simulink model "Drone_NAV_SLAM"  (R2024a)
settings: Solver=FixedStepAuto  StartTime=0.0  StopTime=inf  FixedStep=0.05  RelTol=1e-3
undefined symbols (not defined in the file): DiscIntNeverNeededParam, gray
libraries: robotcorelib x5, mspfiltlib x1, visiongeotforms x1
settings Model: Creator=quentinlandon  LastModifiedBy=quentinlandon
settings SolverCC: AllowMultiTaskInputOutput=on  ConcurrentTasks=on
settings SFSimCC: SimTargetLang=C++

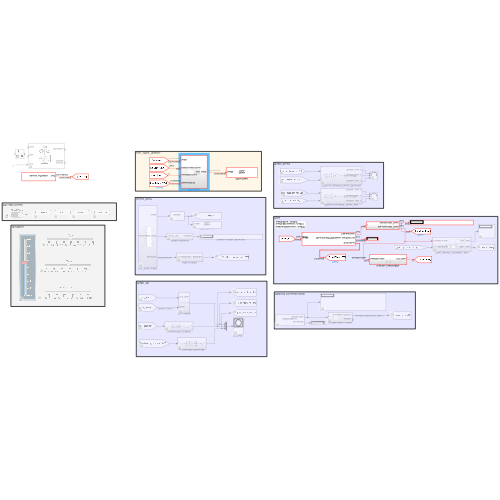
[thumbnail: Simulink's stored preview of the top-level diagram]
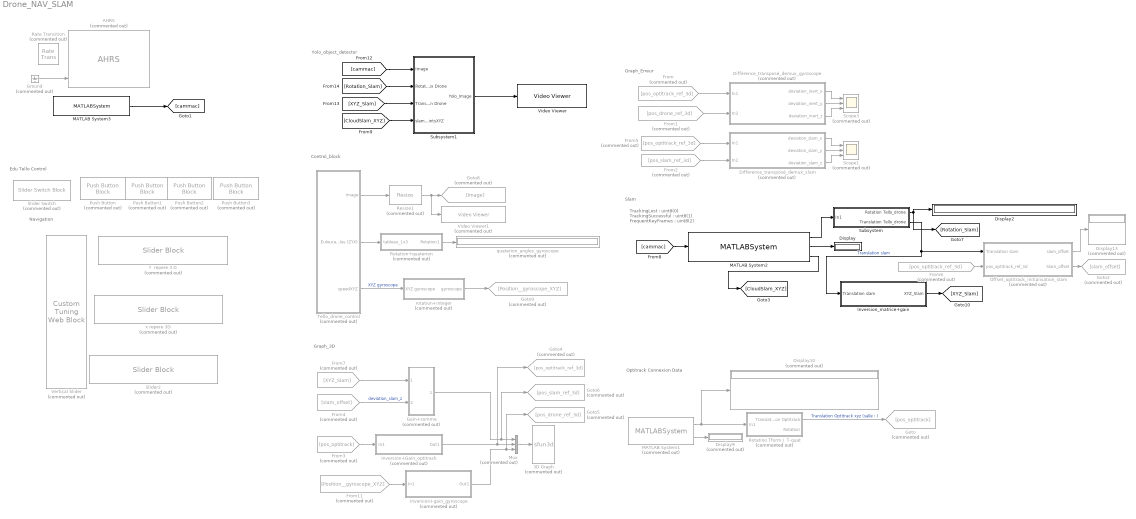
== system Drone_NAV_SLAM ==
  note: Control_block
  note: Graph_Erreur
  note: Graph_3D
  note: Slam
  note: Yolo_object_detector
  note: Optitrack Connexion Data
  note: TrackingLost : uint8(0)
      | TrackingSuccessful : uint8(1)
      | FrequentKeyFrames : uint8(2)
  note: Navigation
  note: Edu Tello Control
  3D Graph : S-Function  Commented=on  LoadFcn=if exist('sfun3d','file'), sfun3d([],[],[],'LoadBlock'); end  FunctionName=sfun3d  Parameters=ax,T,np,cp,gd,ls,mk,mx,hd,tb  SFunctionDeploymentMode=off  EnableBusSupport=off  mask(3D Graph){np=3, ax=[-5 5 -5 5 -5 5], mx=1e4, T=-1, cp=[3 2 1], gd=on, hd=off, tb=on, ls=-, mk=none}
      mask prompts: np "Number of moving points (lines)"; ax "Range: [xmin xmax  ymin ymax zmin zmax]"; mx "Max number of points in each line"; T "Sampling Time"; cp "Camera position (use [0 0 1] for 2D XY view)"; gd "Grid (on|off)"; hd "HeadMarkers (on|off)"; tb "Toolbar (on|off)"; ls "LineStyle"; mk "LineMarker"
      mask help:
      | This block plots the position of several points in the XYZ space. The input contains the coordinates of all the points (x1,y1,z1,x2,y2,z2,...).
      | The number of moving points (lines), the XYZ ranges, sampling time, camera position, and grid (among other things) can be set as mask parameters.
      settings: CopyFcn=if exist('sfun3d','file'), sfun3d([],[],[],'CopyBlock'); end  DeleteFcn=if exist('sfun3d','file'), sfun3d([],[],[],'DeleteBlock'); end  NameChangeFcn=if exist('sfun3d','file'), sfun3d([],[],[],'NameChange'); end
      mask Help:
      | This block plots the position of several points in the XYZ space. The input contains the coordinates of all the points (x1,y1,z1,x2,y2,z2,...).
      | The number of moving points (lines), the XYZ ranges, sampling time, camera position, and grid (among other things) can be set as mask parameters.
      mask TypeOptions ls: - | -- | : | -. | none
      mask TypeOptions mk: none | . | + | o | * | x | square | diamond | v | ^ | > | < | pentagram | hexagram
      mask Display: plot([.05 .95 .95 .05 .05],[.45 .45 .95 .95 .45], 0.5+cos(0:0.1:2*pi)*0.3,0.7+sin(0:0.1:2*pi)*0.2)
  AHRS : mspfiltlib/AHRS  Commented=on  DispRefFrame=NED  DecimationFactor=1  InitialProcessNoise=ahrsfilter.defaultProcessNoise  OrientationFormat=quaternion  SimulateUsing=Interpreted execution  AccelerometerNoise=0.0001924722  GyroscopeNoise=9.1385e-5  MagnetometerNoise=0.1  GyroscopeDriftNoise=3.0462e-13  LinearAccelerationNoise=0.0096236100000000012  MagneticDisturbanceNoise=0.5  LinearAccelerationDecayFactor=0.5  MagneticDisturbanceDecayFactor=0.5  ExpectedMagneticFieldStrength=50
  Différence_transposé_demux_gyroscope : Subsystem  Commented=on
  Différence_transposé_demux_slam : Subsystem  Commented=on
  Display : Display
  Display10 : Display  Commented=on
  Display13 : Display  Commented=on
  Display2 : Display
  Display9 : Display  Commented=on
  From : From  Commented=on  GotoTag=pos_optitrack_ref_3d
  From1 : From  Commented=on  GotoTag=pos_drone_ref_3d
  From11 : From  Commented=on  GotoTag=Position__gyroscope_XYZ
  From2 : From  Commented=on  GotoTag=pos_slam_ref_3d
  From3 : From  Commented=on  GotoTag=pos_optitrack
  From4 : From  Commented=on  GotoTag=slam_offset
  From5 : From  Commented=on  GotoTag=pos_optitrack_ref_3d
  From6 : From  Commented=on  GotoTag=pos_optitrack_ref_3d
  From7 : From  Commented=on  GotoTag=XYZ_Slam
  Gain+somme : Subsystem  Commented=on
  Goto : Goto  Commented=on  GotoTag=pos_optitrack
  Goto2 : Goto  Commented=on  GotoTag=slam_offset
  Goto4 : Goto  Commented=on  GotoTag=pos_optitrack_ref_3d
  Goto5 : Goto  Commented=on  GotoTag=pos_drone_ref_3d
  Goto6 : Goto  Commented=on  GotoTag=pos_slam_ref_3d
  Goto8 : Goto  Commented=on  GotoTag=Image
  Goto9 : Goto  Commented=on  GotoTag=Position__gyroscope_XYZ
  Ground : Ground  Commented=on
  Inversion+Gain_optitrack : Subsystem  Commented=on
  Inversion+gain_gyroscope : Subsystem  Commented=on
  Inversion_matrice+gain : Subsystem
  MATLAB System1 : MATLABSystem  Commented=on  System=OptilinkSystem  HostIP=127.0.0.1  ClientIP=127.0.0.1  SimulateUsing=Interpreted execution
      mask Type: OptilinkSystem
      mask Display:
      | disp('OptilinkSystem');
      | port_label('output',1,'Drones data');
      | port_label('output',2,'Connected');
  MATLAB System2 : MATLABSystem  System=MonoVisualSLAMSystem  FocalLength=[1002.77, 1006.3]  PrincipalPoint=[ 640.67, 365.61 ]  ImageSize=[ 720, 1280 ]  ScaleFactor=1.1  NumLevels=6  MaxNumPoints=1000  SkipMaxFrames=1  TrackFeatureRange=[ 50, 120 ]  LoopClosureThreshold=50  Verbose=false  ThreadLevel=8  SimulateUsing=Interpreted execution
      mask Type: MonoVisualSLAMSystem
      mask Display:
      | disp('MonoVisualSLAMSystem');
      | port_label('input',1,'Image');
      | port_label('output',1,'Camera Pose');
      | port_label('output',2,'Tracking Lost');
      | port_label('output',3,'XYZ Points');
  MATLAB System3 : MATLABSystem  System=camera_ordinateur  SimulateUsing=Interpreted execution
      mask Type: camera_ordinateur
      mask Display:
      | disp('camera_ordinateur');
      | port_label('output',1,'img');
  Mux : Mux  Commented=on  Inputs=3
  Offset_optitrack_initialisation_slam : Subsystem  Commented=on
  Push Button : PushButtonBlock  Commented=on  ButtonText=Takeoff  OffValue=0.000000
  Push Button1 : PushButtonBlock  Commented=on  ButtonText=Land  OffValue=0.000000
  Push Button2 : PushButtonBlock  Commented=on  ButtonText=MoveXYZ  OffValue=0.000000
  Push Button3 : PushButtonBlock  Commented=on  ButtonText=Moverotate  OffValue=0.000000
  Rate Transition : RateTransition  Commented=on
  Resize1 : visiongeotforms/Resize  Commented=on  specify=Output size as a percentage of input size  rfactor=[50 50]  outCols=25  outRows=25  outRowsCols=[25 35]  interp_method=Bilinear  antialias=on  useROI=off  roiFlag=off  roundingMode=Nearest  overflowMode=on  prodOutputMode=Binary point scaling  prodOutputWordLength=32  prodOutputFracLength=10
  Rotatino Tform /  T-quat : Subsystem  Commented=on
  Rotation+quaterion : Subsystem  Commented=on
  Scope1 : Scope  Commented=on  NumInputPorts=3
  Scope3 : Scope  Commented=on  NumInputPorts=3
  Slider Switch : SliderSwitchBlock  Commented=on
      settings: Values={{'Off', 'On'}, [0 1]}
  Slider2 : SliderBlock  Commented=on  ScaleMin=-180  ScaleMax=180
  Subsystem : Subsystem
  Subsystem1 : Subsystem
  Tello_drone_control : Subsystem  Commented=on
  Vertical Slider : CustomTuningWebBlock  Commented=on  LabelPosition=Hide  ShowInitialText=on  Configuration="{\"components\":[{\"name\":\"LinearScaleComponent\",\"settings\":{\"bounds\":{\"max\":2,\"min\":-2,\"tickInterval\":\"auto\"},\"internalTickHeightScaleFactor\":0.5,\"labelColor\":[255,255,200],\"labelFont\":{\"font\":\"Arial\",\"fontSize\":12},\"labelOffset\":0.05,\"labelTransparency\":1,\"needleImage\":{\"size\":[596,842],\"src\":\"data:image\\/svg+xml;base64,PD94bWwgdmVyc2lvbj0iMS4wIiBlbmNvZGluZz0idXRmLTgiPz4NCjwhLS0gR2VuZXJhdG9yOiBBZG9iZSBJbGx1c3RyYXRvciAyNS4wLjAsIFNWRyBFeHBvcnQgUGx1Zy1JbiAuIFNWRyBWZXJzaW9uOiA2LjAwIEJ1aWxkIDApICAtLT4NCjxzdmcgdmVyc2lvbj0iMS4xIg0KCSBpZD0ic3ZnOCIgeG1sbnM6Y2M9Imh0dHA6Ly9jcmVhdGl2ZWNvbW1vbnMub3JnL25zIyIgeG1sbnM6ZGM9Imh0dHA6Ly9wdXJsLm9yZy9kYy9lbGVtZW50cy8xLjEvIiB4bWxuczppbmtzY2FwZT0iaHR0cDovL3d3dy5pbmtzY2FwZS5vcmcvbmFtZXNw ...(+2420 chars)\",\"srcOrientation\":\"horizontal\"},\"needleOffset\":[0.0642123287671233,-0.8044596912521441],\"needleSize\":{\"height\":0.07668067226890757,\"width\":0.4337797619047619},\"position\":[0.03623949579831933,0.2829861111111111,0.6088789682539683,0.9196428571428571],\"referencePoint\":\"auto\",\"scaleColors\":[],\"scaleColorsSize\":0.2,\"scaleDirection\":\"BT\",\"showLabels\":1,\"showMinorTicks\":0,\"showSpanLine\":1,\"showTicks\":1,\"tickColor\":[252,252,197],\"tickTransparency\":1,\"valueBarColor\":[0,114,189],\"valueBarOffset\":-0.27,\"valueBarSize\":0.1,\"valueBarTransparency\":1}},{\"name\":\"BackgroundImageComponent\",\"settings\":{\"image\":{\"size\":[380,101],\"src\":\"data:image\\/svg+xml;base64,PHN2ZyB4bWxucz0iaHR0cDovL3d3dy53My5vcmcvMjAwMC9zdmciIHhtbG5zOnhsaW5rPSJodHRwOi8vd3d3LnczLm9yZy8xOTk5L3hsaW5rIiB2aWV3Qm94PSIwIDAgMzgwIDEwMSI+PGRlZnM+PHN0eWxlPi5jbHMtMXtmaWxsOiMwMDJiNDI7fS5jbHMtMntmaWxsOiM0MjcwODI7fS5jbHMtM3tmaWxsOnVybCgjcmFkaWFsLWdyYWRpZW50KTt9LmNscy00e2ZpbGw6I2M4YzhjODtzdHJva2U6IzAwMDt9PC9zdHlsZT48cmFkaWFsR3JhZGllbnQgaWQ9InJhZGlhbC1ncmFkaWVudCIgY3g9IjE5MCIgY3k9IjUwLjUiIHI9IjI2OS4yMSIgZ3JhZGllbnRVbml0cz0idXNlclNwYWNlT25Vc2UiPjxzdG9wIG9mZnNldD0iMC4wMSIgc3RvcC1jb2xvcj0iIzNlNGY1OCIvPjxzdG9wIG9mZnNldD0iMC4wNiIgc3RvcC1jb2xvcj0iIzQ0NTc2MSIvPjxzdG9wIG9mZnNldD0iMC4xNSIgc3RvcC1jb2xvcj0iIzU1NmE3NiIvPjxzdG9wIG9mZnNldD0iMC4yNSIgc3RvcC1jb2xvcj0iIzZkODg5NSIvPjxzdG9wIG9mZnNldD0iMC4zOCIgc3RvcC1jb2xvcj0iIzhmYjJjMyIvPjxzdG9wIG9mZnNldD0iMC41MiIgc3RvcC1jb2xvcj0iI2I2ZTRmYSIvPjxzdG9wIG9mZnNldD0iMSIgc3RvcC1jb2xvcj0iIzE1NDY1NyIvPjwvcmFkaWFsR3JhZGllbnQ+PC9kZWZzPjxnIGlkPSJmcmFtZSI+PGcgaWQ9IkxheWVyXzIiIGRhdGEtbmFtZT0iTGF5ZXIgMiI+PGcgaWQ9IkxheWVyXzEtMiIgZGF0YS1uYW1lPSJMYXllciAxLTIiPjxyZWN0IGlkPSJyZWN0MTAzNiIgY2xhc3M9ImNscy0xIiB4PSIxMSIgeT0iMTEiIHdpZHRoPSIzNTgiIGhlaWdodD0iNzkiLz48cGF0aCBpZD0icGF0aDEwMzgiIGNsYXNzPSJjbHMtMiIgZD0iTTgsOFY5M0gzNzJWOFpNMzY5LDkwSDExVjExSDM2OVoiLz48cGF0aCBpZD0icGF0aDEwNDAiIGNsYXNzPSJjbHMtMyIgZD0iTTAsMFYxMDFIMzgwVjBaTTM3Miw5M0g4VjhIMzcyWiIvPjwvZz48L2c+PC9nPjxnIGlkPSJ0cmFjayI+PHBhdGggaWQ9InJlY3QxNjExIiBjbGFzcz0iY2xzLTQiIGQ9Ik0zMy4zNywyNi41OUgzNDYuNjNjNCwwLDcuMjUsMi42LDcuMjUsNS44MWgwYzAsMy4yMS0zLjI1LDUuODItNy4yNSw1LjgySDMzLjM3Yy00LDAtNy4yNS0yLjYxLTcuMjUtNS44MmgwQzI2LjEyLDI5LjE5LDI5LjM3LDI2LjU5LDMzLjM3LDI2LjU5WiIvPjwvZz48L3N2Zz4=\",\"srcOrientation\":\"horizontal\"},\"position\":[0,0,1,1],\"scaleMode\":\"0\"}},{\"name\":\"ForegroundImageComponent\",\"settings\":{\"image\":{\"size\":[0,0],\"src\":\"default\",\"srcOrientation\":[]},\"isForeground\":1,\"position\":[0,0,1,1],\"scaleMode\":\"0\"}}],\"settings\":{\"BindingType\":\"param\",\"aspectRatio\":3.7777777777777777,\"backgroundColor\":[0,0,0,\"1\"],\"backgroundOffset\":0,\"backgroundOpacity\":1,\"fixedAspectRatio\":\"on\",\"foregroundColor\":[252,252,196],\"orientation\":\"vertical\",\"showBackgroundColor\":false,\"value\":0,\"version\":\"R2023a\"},\"type\":\"LinearGauge\"}"
  Video Viewer : VideoViewer  colormapValue=gray(256)  FigPos=[1 642 730 455]
  Video Viewer1 : VideoViewer  Commented=on  FigPos=[269 662 902 426]
  Y  repere 3 D : SliderBlock  Commented=on  ScaleMin=-2  ScaleMax=2
  quaterion_angles_gyroscope : Display  Commented=on
  rotation+integer : Subsystem  Commented=on
  x repere 3D : SliderBlock  Commented=on  ScaleMin=-2  ScaleMax=2
  wires:
  MATLAB System2/2 -> Display/1
  Subsystem/1(Rotation Tello_drone) -> Display2/1, [Rotation_Slam]
  MATLAB System1/2 -> Display9/1
  MATLAB System1/1 -> Display10/1, Rotatino Tform /  T-quat/1(In1)
  Subsystem/2(Translation Tello_drone) -> Offset_optitrack_initialisation_slam/1(Translation slam), Inversion_matrice+gain/1(Translation slam)  "Translation slam"
  Tello_drone_control/3(speedXYZ) -> rotation+integer/1(XYZ gyroscope)  "XYZ gyroscope"
  Rotatino Tform /  T-quat/1(Translation Optitrack) -> Goto/1  "Translation Optitrack xyz (salle : )"
  Tello_drone_control/2(Euleurangles (ZYX)) -> Rotation+quaterion/1(tableau_1x3)
  Rotation+quaterion/1(Rotation1) -> quaterion_angles_gyroscope/1
  Resize1/1 -> Goto8/1, Video Viewer1/1
  Tello_drone_control/1(Image) -> Resize1/1
  rotation+integer/1(gyroscope) -> Goto9/1
  Offset_optitrack_initialisation_slam/1(slam_offset) -> Display13/1
  Inversion_matrice+gain/1(XYZ_Slam) -> [XYZ_Slam]
  Offset_optitrack_initialisation_slam/2(Slam_offset) -> Goto2/1
  From6/1 -> Offset_optitrack_initialisation_slam/2(pos_optitrack_ref_3d)
  Mux/1 -> 3D Graph/1
  MATLAB System2/1 -> Subsystem/1(In1)
  Ground/1 -> AHRS/3
  From7/1 -> Gain+somme/1(XYZ_Slam)
  From4/1 -> Gain+somme/2(Offset)  "deviation_slam_z"
  Inversion+Gain_optitrack/1(Out1) -> Goto4/1, Mux/2
  From3/1 -> Inversion+Gain_optitrack/1(In1)
  Inversion+gain_gyroscope/1(Out1) -> Goto5/1, Mux/3
  From11/1 -> Inversion+gain_gyroscope/1(In1)
  Gain+somme/1(Out1) -> Goto6/1, Mux/1
  From/1 -> Différence_transposé_demux_gyroscope/1(In1)
  From1/1 -> Différence_transposé_demux_gyroscope/2(In2)
  Différence_transposé_demux_gyroscope/1(deviation_inert_x) -> Scope3/1
  Différence_transposé_demux_gyroscope/2(deviation_inert_y) -> Scope3/2
  Différence_transposé_demux_gyroscope/3(deviation_inert_z) -> Scope3/3
  From5/1 -> Différence_transposé_demux_slam/1(In1)
  From2/1 -> Différence_transposé_demux_slam/2(In2)
  Différence_transposé_demux_slam/1(deviation_slam_x) -> Scope1/1
  Différence_transposé_demux_slam/2(deviation_slam_y) -> Scope1/2
  Différence_transposé_demux_slam/3(deviation_slam_z) -> Scope1/3
  [cammac] -> MATLAB System2/1
  MATLAB System3/1 -> [cammac]
  Subsystem1/1(Yolo_Image) -> Video Viewer/1
  [cammac] -> Subsystem1/1(Image)
  [XYZ_Slam] -> Subsystem1/3(Translation Drone)
  [Rotation_Slam] -> Subsystem1/2(Rotation matrix Drone)
  MATLAB System2/3 -> [CloudSlam_XYZ]
  [CloudSlam_XYZ] -> Subsystem1/4(slamPointsXYZ)

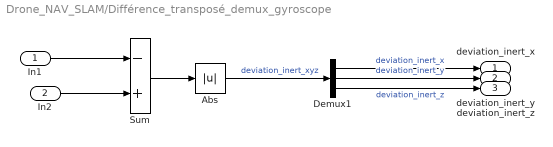
== system Drone_NAV_SLAM/Différence_transposé_demux_gyroscope ==
  In1 : Inport
  In2 : Inport  Port=2
  Abs : Abs  SaturateOnIntegerOverflow=off
  Demux1 : Demux  Outputs=3
  Sum : Sum  Inputs=-+
  deviation_inert_x : Outport
  deviation_inert_y : Outport  Port=2
  deviation_inert_z : Outport  Port=3
  wires:
  Demux1/3 -> deviation_inert_z/1  "deviation_inert_z"
  Demux1/2 -> deviation_inert_y/1  "deviation_inert_y"
  In2/1 -> Sum/2
  In1/1 -> Sum/1
  Demux1/1 -> deviation_inert_x/1  "deviation_inert_x"
  Abs/1 -> Demux1/1  "deviation_inert_xyz"
  Sum/1 -> Abs/1

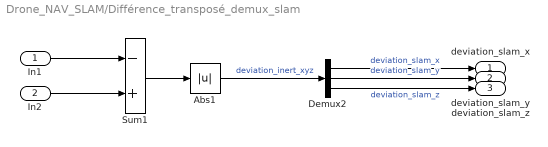
== system Drone_NAV_SLAM/Différence_transposé_demux_slam ==
  In1 : Inport
  In2 : Inport  Port=2
  Abs1 : Abs  SaturateOnIntegerOverflow=off
  Demux2 : Demux  Outputs=3
  Sum1 : Sum  Inputs=-+
  deviation_slam_x : Outport
  deviation_slam_y : Outport  Port=2
  deviation_slam_z : Outport  Port=3
  wires:
  In1/1 -> Sum1/1
  Demux2/1 -> deviation_slam_x/1  "deviation_slam_x"
  In2/1 -> Sum1/2
  Demux2/3 -> deviation_slam_z/1  "deviation_slam_z"
  Abs1/1 -> Demux2/1  "deviation_inert_xyz"
  Sum1/1 -> Abs1/1
  Demux2/2 -> deviation_slam_y/1  "deviation_slam_y"

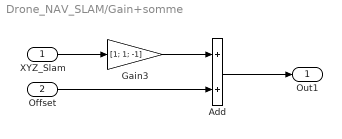
== system Drone_NAV_SLAM/Gain+somme ==
  XYZ_Slam : Inport
  Offset : Inport  Port=2
  Add : Sum
  Gain3 : Gain  Gain=[1; 1; -1]
  Out1 : Outport
  wires:
  XYZ_Slam/1 -> Gain3/1
  Offset/1 -> Add/2
  Add/1 -> Out1/1
  Gain3/1 -> Add/1

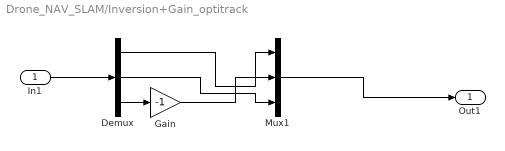
== system Drone_NAV_SLAM/Inversion+Gain_optitrack ==
  In1 : Inport
  Demux : Demux  Outputs=3
  Gain : Gain  Gain=-1
  Mux1 : Mux  Inputs=3
  Out1 : Outport
  wires:
  Mux1/1 -> Out1/1
  Demux/3 -> Gain/1
  Demux/2 -> Mux1/3
  In1/1 -> Demux/1
  Demux/1 -> Mux1/1
  Gain/1 -> Mux1/2

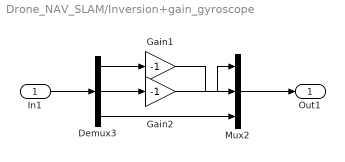
== system Drone_NAV_SLAM/Inversion+gain_gyroscope ==
  In1 : Inport
  Demux3 : Demux  Outputs=3
  Gain1 : Gain  Gain=-1
  Gain2 : Gain  Gain=-1
  Mux2 : Mux  Inputs=3
  Out1 : Outport
  wires:
  In1/1 -> Demux3/1
  Mux2/1 -> Out1/1
  Demux3/1 -> Gain1/1
  Demux3/3 -> Mux2/3
  Gain1/1 -> Mux2/2
  Demux3/2 -> Gain2/1
  Gain2/1 -> Mux2/1

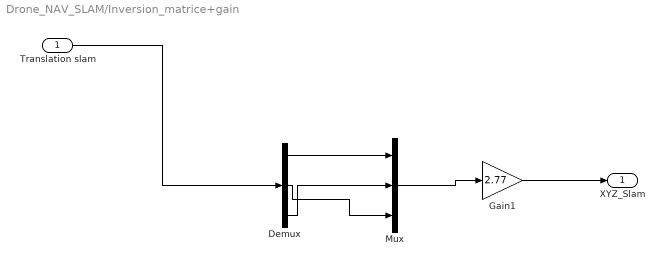
== system Drone_NAV_SLAM/Inversion_matrice+gain ==
  Translation slam : Inport
  Demux : Demux  Outputs=3
  Gain1 : Gain  Gain=2.77
  Mux : Mux  Inputs=3
  XYZ_Slam : Outport
  wires:
  Translation slam/1 -> Demux/1
  Gain1/1 -> XYZ_Slam/1
  Demux/1 -> Mux/1
  Demux/3 -> Mux/2
  Demux/2 -> Mux/3
  Mux/1 -> Gain1/1

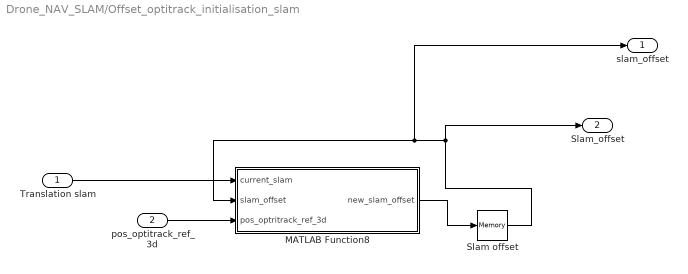
== system Drone_NAV_SLAM/Offset_optitrack_initialisation_slam ==
  Translation slam : Inport
  pos_optitrack_ref_3d : Inport  Port=2
  MATLAB Function8 : MATLAB Function  TreatAsAtomicUnit=on
  Slam offset : Memory  InitialCondition=[0;0;0]
  slam_offset : Outport
  Slam_offset : Outport  Port=2
  wires:
  MATLAB Function8/1(new_slam_offset) -> Slam offset/1
  Slam offset/1 -> Slam_offset/1, slam_offset/1, MATLAB Function8/2(slam_offset)
  Translation slam/1 -> MATLAB Function8/1(current_slam)
  pos_optitrack_ref_3d/1 -> MATLAB Function8/3(pos_optritrack_ref_3d)

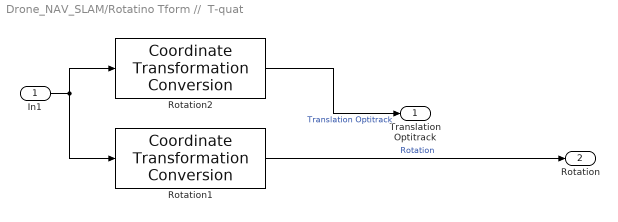
== system Drone_NAV_SLAM/Rotatino Tform //  T-quat ==
  In1 : Inport
  Rotation1 : robotcorelib/Coordinate Transformation Conversion  InputRepresentation=Homogeneous Transformation  InputEulerSequence=ZYX  ShowTrVecInputPort=on  OutputRepresentation=Quaternion  OutputEulerSequence=ZYX  ShowTrVecOutputPort=off  SimulateUsing=Code generation
      settings: LibrarySourceBlock=uavutilslib/Coordinate Transformation Conversion
  Rotation2 : robotcorelib/Coordinate Transformation Conversion  InputRepresentation=Homogeneous Transformation  InputEulerSequence=ZYX  ShowTrVecInputPort=on  OutputRepresentation=Translation Vector  OutputEulerSequence=ZYX  ShowTrVecOutputPort=off  SimulateUsing=Code generation
      settings: LibrarySourceBlock=uavutilslib/Coordinate Transformation Conversion
  Translation Optitrack : Outport
  Rotation : Outport  Port=2
  wires:
  Rotation1/1 -> Rotation/1  "Rotation"
  Rotation2/1 -> Translation Optitrack/1  "Translation Optitrack"
  In1/1 -> Rotation2/1, Rotation1/1

== system Drone_NAV_SLAM/Rotation+quaterion ==
  tableau_1x3 : Inport
  Rotation : robotcorelib/Coordinate Transformation Conversion  InputRepresentation=Euler Angles  InputEulerSequence=ZYX  ShowTrVecInputPort=on  OutputRepresentation=Quaternion  OutputEulerSequence=ZYX  ShowTrVecOutputPort=off  SimulateUsing=Code generation
      settings: LibrarySourceBlock=uavutilslib/Coordinate Transformation Conversion
  Transpose : Math  Operator=transpose
  Rotation1 : Outport
  wires:
  Rotation/1 -> Rotation1/1  "Rotation"
  Transpose/1 -> Rotation/1
  tableau_1x3/1 -> Transpose/1

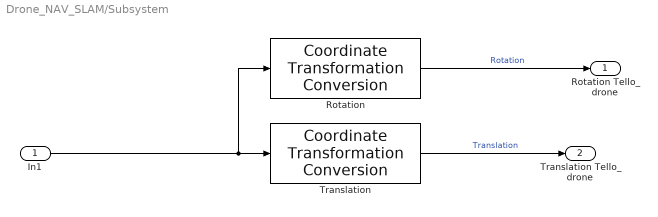
== system Drone_NAV_SLAM/Subsystem ==
  In1 : Inport
  Rotation : robotcorelib/Coordinate Transformation Conversion  InputRepresentation=Homogeneous Transformation  InputEulerSequence=ZYX  ShowTrVecInputPort=on  OutputRepresentation=Rotation Matrix  OutputEulerSequence=ZYX  ShowTrVecOutputPort=off  SimulateUsing=Code generation
      settings: LibrarySourceBlock=uavutilslib/Coordinate Transformation Conversion
  Translation : robotcorelib/Coordinate Transformation Conversion  InputRepresentation=Homogeneous Transformation  InputEulerSequence=ZYX  ShowTrVecInputPort=on  OutputRepresentation=Translation Vector  OutputEulerSequence=ZYX  ShowTrVecOutputPort=on  SimulateUsing=Code generation
      settings: LibrarySourceBlock=uavutilslib/Coordinate Transformation Conversion
  Rotation Tello_drone : Outport
  Translation Tello_drone : Outport  Port=2
  wires:
  Translation/1 -> Translation Tello_drone/1  "Translation"
  Rotation/1 -> Rotation Tello_drone/1  "Rotation"
  In1/1 -> Rotation/1, Translation/1

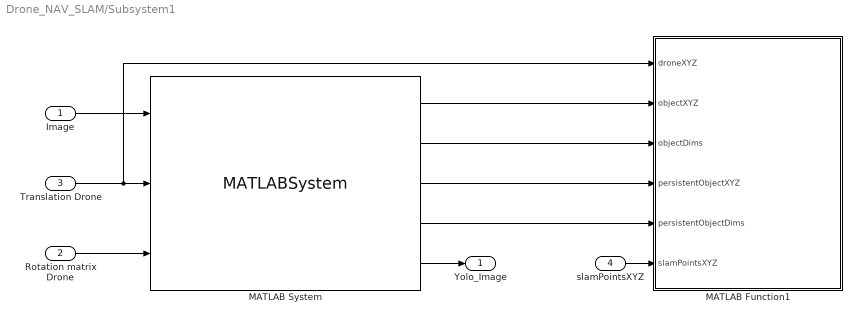
== system Drone_NAV_SLAM/Subsystem1 ==
  Image : Inport
  Rotation matrix Drone : Inport  Port=2
  Translation Drone : Inport  Port=3
  slamPointsXYZ : Inport  Port=4
  MATLAB Function1 : MATLAB Function  TreatAsAtomicUnit=on
  MATLAB System : MATLABSystem  System=Yolo_Object_Detector  SimulateUsing=Interpreted execution
      mask Type: Yolo_Object_Detector
      mask Display:
      | disp('Yolo_Object_Detector');
      | port_label('input',1,'Image');
      | port_label('input',2,'TranslationMatrix');
      | port_label('input',3,'RotationMatrix');
      | port_label('output',1,'ObjectXYZ');
      | port_label('output',2,'ObjectDims');
      | port_label('output',3,'PersistentObjectXYZ');
      | port_label('output',4,'PersistentObjectDims');
      | port_label('output',5,'AnnotatedImage');
  Yolo_Image : Outport
  wires:
  Image/1 -> MATLAB System/1
  Translation Drone/1 -> MATLAB Function1/1(droneXYZ), MATLAB System/2
  MATLAB System/3 -> MATLAB Function1/4(persistentObjectXYZ)
  MATLAB System/4 -> MATLAB Function1/5(persistentObjectDims)
  MATLAB System/2 -> MATLAB Function1/3(objectDims)
  slamPointsXYZ/1 -> MATLAB Function1/6(slamPointsXYZ)
  MATLAB System/5 -> Yolo_Image/1
  Rotation matrix Drone/1 -> MATLAB System/3
  MATLAB System/1 -> MATLAB Function1/2(objectXYZ)

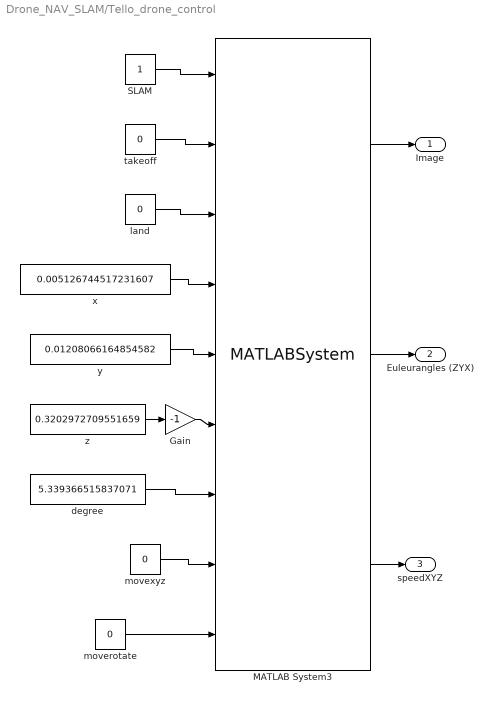
== system Drone_NAV_SLAM/Tello_drone_control ==
  Gain : Gain  Gain=-1
  MATLAB System3 : MATLABSystem  System=Tello_drone_control  droneIP=193.169.0.11  SimulateUsing=Interpreted execution
      mask Type: Tello_drone_control
      mask Display:
      | disp('Tello_drone_control');
      | port_label('input',1,'Slam');
      | port_label('input',2,'tkoff');
      | port_label('input',3,'landing');
      | port_label('input',4,'xMove');
      | port_label('input',5,'yMove');
      | port_label('input',6,'zMove');
      | port_label('input',7,'degree');
      | port_label('input',8,'movexyz');
      | port_label('input',9,'moverotate');
      | port_label('output',1,'imgresize');
      | port_label('output',2,'Eulerangles');
      | port_label('output',3,'speedXYZ');
  SLAM : Constant
  degree : Constant  Value=5.339366515837071
  land : Constant  Value=0
  moverotate : Constant  Value=0
  movexyz : Constant  Value=0
  takeoff : Constant  Value=0
  x : Constant  Value=0.005126744517231607
  y : Constant  Value=0.01208066164854582
  z : Constant  Value=0.3202972709551659
  Image : Outport
  Euleurangles (ZYX) : Outport  Port=2
  speedXYZ : Outport  Port=3
  wires:
  moverotate/1 -> MATLAB System3/9
  land/1 -> MATLAB System3/3
  y/1 -> MATLAB System3/5
  x/1 -> MATLAB System3/4
  Gain/1 -> MATLAB System3/6
  z/1 -> Gain/1
  degree/1 -> MATLAB System3/7
  SLAM/1 -> MATLAB System3/1
  movexyz/1 -> MATLAB System3/8
  MATLAB System3/1 -> Image/1
  takeoff/1 -> MATLAB System3/2
  MATLAB System3/2 -> Euleurangles (ZYX)/1
  MATLAB System3/3 -> speedXYZ/1

== system Drone_NAV_SLAM/rotation+integer ==
  XYZ gyroscope : Inport
  Discrete-Time Integrator : DiscreteIntegrator  SampleTime=-1  ICPrevOutput=DiscIntNeverNeededParam  ICPrevScaledInput=DiscIntNeverNeededParam
  Transpose : Math  Operator=transpose
  gyroscope : Outport
  wires:
  XYZ gyroscope/1 -> Discrete-Time Integrator/1
  Transpose/1 -> gyroscope/1  "gyroscope"
  Discrete-Time Integrator/1 -> Transpose/1

== matlab function Drone_NAV_SLAM/Subsystem1/MATLAB Function1 ==
  data: droneXYZ input; objectXYZ input; objectDims input; persistentObjectXYZ input; persistentObjectDims input; slamPointsXYZ input
function plotCubes(droneXYZ, objectXYZ, objectDims, persistentObjectXYZ, persistentObjectDims, slamPointsXYZ)
    %#codegen
    coder.extrinsic('figure', 'clf', 'hold', 'patch', 'xlabel', 'ylabel', 'zlabel', 'grid', 'axis', 'title', 'view', 'xlim', 'ylim', 'zlim');
    
    %% Initialisation de la figure
    fig = figure(1);
    clf(fig); % Effacer la figure courante
    hold on;
    
    %% Tracer la position du drone
    plot3(droneXYZ(1), droneXYZ(2), droneXYZ(3), 'ro', 'MarkerSize', 10, 'LineWidth', 2);
    
    %% Tracer les objets détectés
    for i = 1:size(objectXYZ, 1)
        if all(objectXYZ(i, :) ~= 0)
            plotBox3D(objectXYZ(i, :), objectDims(i, :), [1, 0, 0], 0.3);
        end
    end
    
    %% Tracer les objets persistants
    for i = 1:size(persistentObjectXYZ, 1)
        if all(persistentObjectXYZ(i, :) ~= 0)
            plotBox3D(persistentObjectXYZ(i, :), persistentObjectDims(i, :), [0, 1, 0], 0.3);
        end
    end
    
    %% Tracer les points générés par le SLAM
    if ~isempty(slamPointsXYZ)
        plot3(slamPointsXYZ(:, 1), slamPointsXYZ(:, 2), slamPointsXYZ(:, 3), 'bo', 'MarkerSize', 1, 'LineWidth', 1);
    end

    %% Paramètres d'affichage du graphique
    xlabel('X');
    ylabel('Y');
    zlabel('Z');
    grid on;
    axis equal;
    title('Drone and Detected Objects Positions');
    view(3); % Vue en 3D
    
    % Fixer les limites des axes
    xlim([-5, 5]);
    ylim([-5, 5]);
    zlim([0, 2]);
    
    hold off;
end

function plotBox3D(center, dims, color, alpha)
    coder.extrinsic('patch');

    % Calculer les coins de la boite englobante
    corners = [
        -dims(1)/2, -dims(2)/2, -dims(3)/2;
        dims(1)/2, -dims(2)/2, -dims(3)/2;
        dims(1)/2, dims(2)/2, -dims(3)/2;
        -dims(1)/2, dims(2)/2, -dims(3)/2;
        -dims(1)/2, -dims(2)/2, dims(3)/2;
        dims(1)/2, -dims(2)/2, dims(3)/2;
        dims(1)/2, dims(2)/2, dims(3)/2;
        -dims(1)/2, dims(2)/2, dims(3)/2;
    ];

    % Déplacer les coins vers la position centrale de l'objet
    corners = corners + center;

    % Faces du cube
    faces = [
        1 2 3 4;
        2 6 7 3;
        6 5 8 7;
        5 1 4 8;
        4 3 7 8;
        1 5 6 2;
    ];

    % Tracer les faces du cube
    for i = 1:size(faces, 1)
        patch('Vertices', corners, 'Faces', faces(i, :), 'FaceColor', color, 'FaceAlpha', alpha);
    end
end

== matlab function Drone_NAV_SLAM/Offset_optitrack_initialisation_slam/MATLAB Function8 ==
  data: current_slam input; new_slam_offset output; slam_offset input; pos_optritrack_ref_3d input
function new_slam_offset = fcn(current_slam,slam_offset, pos_optritrack_ref_3d)

% If the slam started, and the Offset has not been set yet, assign the
% current Optitrack position 
if (any(current_slam) && ~any(slam_offset))
    new_slam_offset = pos_optritrack_ref_3d;
else
    new_slam_offset = slam_offset;
end 


%new_slam_offset(3) = 0;
